simulink model "SystemLoopDiscrete2022"  (R2022b)
settings: Solver=FixedStepAuto  StartTime=0.0  StopTime=50  RelTol=1e-3  EnableMultiTasking=on
values from neighbouring files (symbols this model uses):
  L = 8.2*10^(-3)    (= 0.0082)    [phaseplane.m]
undefined symbols (not defined in the file or in its folder): Ad, Bd, Cd, Dd, ki, Kp, Ts
libraries: mbedblockslib x3, stm_qeplib x1
settings Model: ExtModeTrigDuration=10  Creator=Marco  LastModifiedBy=Marco
settings OptimizationCC: ReuseModelBlockBuffer=on  EnhancedBackFolding=on  PassReuseOutputArgsAs=Individual arguments  ZeroExternalMemoryAtStartup=off  ZeroInternalMemoryAtStartup=off  MaxStackSize=64  OptimizeBlockOrder=speed  DifferentSizesBufferReuse=on  OptimizationCustomize=off  EfficientTunableParamExpr=on
settings DebuggingCC: ParameterTunabilityLossMsg=error
settings HardwareCC: ProdBitPerPointer=32  ProdBitPerSizeT=32  ProdBitPerPtrDiffT=32  ProdLargestAtomicInteger=Long  ProdLargestAtomicFloat=Double  ProdWordSize=32  ProdLongLongMode=on  ProdHWDeviceType=ARM Compatible->ARM Cortex
settings SFSimCC: MATLABDynamicMemAlloc=off
settings RTWCC: Description=Embedded Coder  SystemTargetFile=ert.tlc  HardwareBoard=STM32 Nucleo F401RE  TemplateMakefile=ert_default_tmf  Toolchain=GNU Tools for ARM Embedded Processors
settings CodeAppCC: ForceParamTrailComments=on  IgnoreCustomStorageClasses=off  OperatorAnnotations=on  SimulinkDataObjDesc=on  SFDataObjDesc=on  InsertBlockDesc=on
settings ERTTargetCC: ExtMode=on  ExtModeTransport=3  ExtModeStaticAlloc=on  ExtModeStaticAllocSize=2000  ExtModeMexFile=ext_xcp  ExtModeMexArgs=1 3 115200  ExtModeIntrfLevel=Level2 - Open

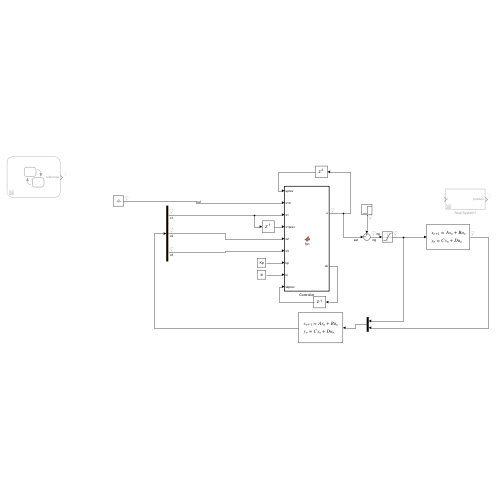
[thumbnail: Simulink's stored preview of the top-level diagram]
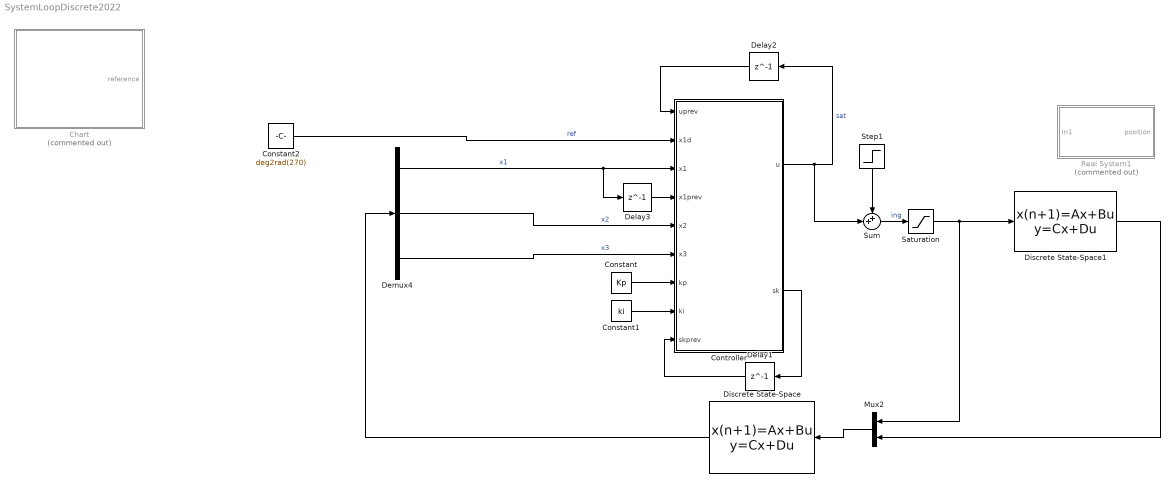
== system SystemLoopDiscrete2022 ==
  Chart : Stateflow chart  Commented=on  TreatAsAtomicUnit=on
  Constant : Constant  Value=Kp  SampleTime=Ts
  Constant1 : Constant  Value=ki  SampleTime=Ts
  Constant2 : Constant  Value=deg2rad(270)
  Controller : MATLAB Function  TreatAsAtomicUnit=on
  Delay1 : Delay  DelayLength=1  InitialCondition=0
  Delay2 : Delay  DelayLength=1  InitialCondition=0
  Delay3 : Delay  DelayLength=1  InitialCondition=0
  Demux4 : Demux  Outputs=3
  Discrete State-Space : DiscreteStateSpace  A=Ad-L*Cd  B=[Bd L]  C=eye(3)  D=[ 0 0; 0 0; 0 0]  SampleTime=Ts
  Discrete State-Space1 : DiscreteStateSpace  A=Ad  B=Bd  C=Cd  D=Dd  SampleTime=Ts
  Mux2 : Mux  Inputs=2
  Real System1 : Subsystem  Commented=on
  Saturation : Saturate  UpperLimit=12  LowerLimit=-12
  Step1 : Step  Time=3  After=1.2  SampleTime=Ts
  Sum : Sum  Inputs=++|
  wires:
  Discrete State-Space/1 -> Demux4/1
  Mux2/1 -> Discrete State-Space/1
  Demux4/2 -> Controller/5(x2)  "x2"
  Step1/1 -> Sum/1
  Sum/1 -> Saturation/1  "ing"
  Discrete State-Space1/1 -> Mux2/2
  Constant/1 -> Controller/7(kp)
  Constant2/1 -> Controller/2(x1d)  "ref"
  Demux4/1 -> Controller/3(x1), Delay3/1  "x1"
  Constant1/1 -> Controller/8(ki)
  Controller/1(u) -> Delay2/1, Sum/2  "sat"
  Demux4/3 -> Controller/6(x3)  "x3"
  Controller/2(sk) -> Delay1/1
  Delay1/1 -> Controller/9(skprev)
  Delay2/1 -> Controller/1(uprev)
  Delay3/1 -> Controller/4(x1prev)
  Saturation/1 -> Discrete State-Space1/1, Mux2/1

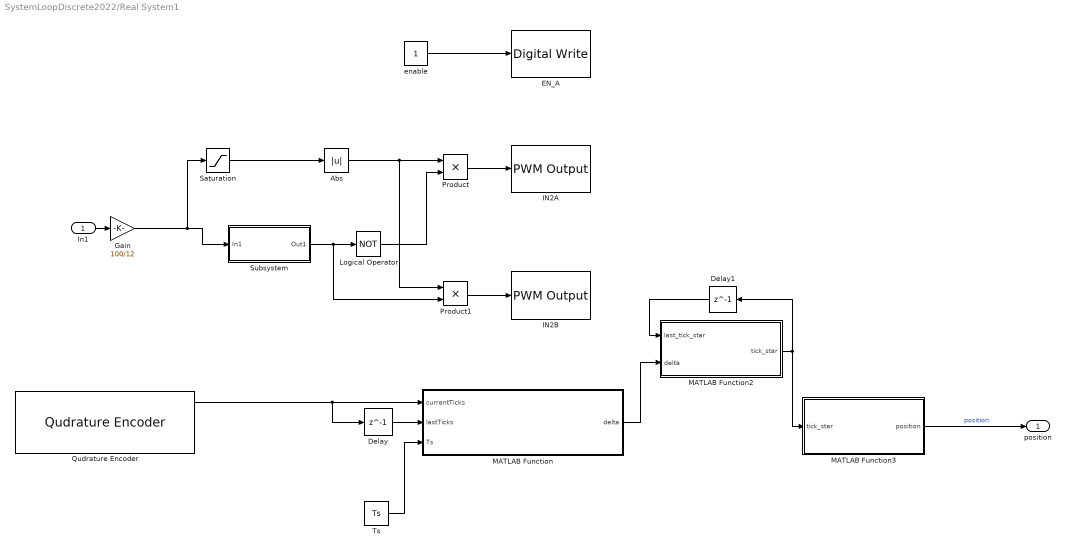
== system SystemLoopDiscrete2022/Real System1 ==
  In1 : Inport
  Abs : Abs  SaturateOnIntegerOverflow=off
  Delay : Delay  DelayLength=1  InitialCondition=0
  Delay1 : Delay  DelayLength=1  InitialCondition=0
  EN_A : mbedblockslib/Digital Write  Pin=2  Direction=output
      settings: LibrarySourceBlock=stmnucleorootlib/Common/Digital Write
  Gain : Gain  Gain=100/12
  IN2A : mbedblockslib/PWM Output  Pin=4  EnableInputFrequency=off  InitialFrequency=PWMFreq  InitialDutyCycle=50  NotificationType=None
      settings: LibrarySourceBlock=stmnucleorootlib/Common/PWM Output
  IN2B : mbedblockslib/PWM Output  Pin=5  EnableInputFrequency=off  InitialFrequency=PWMFreq  InitialDutyCycle=50  NotificationType=None
      settings: LibrarySourceBlock=stmnucleorootlib/Common/PWM Output
  Logical Operator : Logic  Operator=NOT  AllPortsSameDT=off  OutDataTypeStr=boolean
  MATLAB Function : MATLAB Function  TreatAsAtomicUnit=on
  MATLAB Function2 : MATLAB Function  TreatAsAtomicUnit=on
  MATLAB Function3 : MATLAB Function  TreatAsAtomicUnit=on
  Product : Product
  Product1 : Product
  Qudrature Encoder : stm_qeplib/Qudrature Encoder  SampleTime=Ts
  Saturation : Saturate  UpperLimit=100  LowerLimit=-100
  Subsystem : Subsystem
  Ts : Constant  Value=Ts
  enable : Constant
  position : Outport
  wires:
  enable/1 -> EN_A/1
  Subsystem/1(Out1) -> Product1/2, Logical Operator/1
  Saturation/1 -> Abs/1
  Product1/1 -> IN2B/1
  Product/1 -> IN2A/1
  Logical Operator/1 -> Product/2
  Abs/1 -> Product1/1, Product/1
  Gain/1 -> Saturation/1, Subsystem/1(In1)
  MATLAB Function2/1(tick_star) -> MATLAB Function3/1(tick_star), Delay1/1
  Qudrature Encoder/1 -> Delay/1, MATLAB Function/1(currentTicks)
  MATLAB Function/1(delta) -> MATLAB Function2/2(delta)
  Delay1/1 -> MATLAB Function2/1(last_tick_star)
  Ts/1 -> MATLAB Function/3(Ts)
  Delay/1 -> MATLAB Function/2(lastTicks)
  In1/1 -> Gain/1
  MATLAB Function3/1(position) -> position/1  "position"

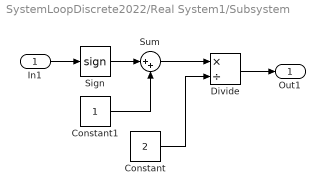
== system SystemLoopDiscrete2022/Real System1/Subsystem ==
  In1 : Inport
  Constant : Constant  Value=2
  Constant1 : Constant
  Divide : Product  Inputs=*/
  Sign : Signum
  Sum : Sum  Inputs=|++
  Out1 : Outport
  wires:
  In1/1 -> Sign/1
  Sign/1 -> Sum/1
  Constant1/1 -> Sum/2
  Sum/1 -> Divide/1
  Constant/1 -> Divide/2
  Divide/1 -> Out1/1

== stateflow chart SystemLoopDiscrete2022/Chart ==
  state Start
    reference = 0;
  state State1
    reference = deg2rad(180)
  state State4
    reference = -180
  state State2
    reference = deg2rad(360)
  state State3
    reference = deg2rad(270)
  state State5
    reference = 0
  (default) -> Start
  Start -> State1 : [after(4,sec)]
  State1 -> State4 : [after(4,sec)]
  State4 -> State2 : [after(4,sec)]
  State3 -> Start : [after(4,sec)]
  State2 -> State5 : [after(4,sec)]
  State5 -> State3 : [after(4,sec)]
  data: reference output

== matlab function SystemLoopDiscrete2022/Controller ==
  data: uprev input; x1d input; x1 input; x1prev input; u output; x2 input; x3 input; kp input; ki input; skprev input; sk output
function [u,sk] = fcn(uprev, x1d, x1, x1prev, x2, x3, kp, ki, skprev)

eprev = x1d-x1prev

stopsumm = ((uprev > 12 & eprev > 0) | (uprev < -12 & eprev < 0));

if ~(stopsumm)
   sk = skprev + eprev
   u = -kp(1)*(x1) - kp(2)*x2 - kp(3)*x3 + ki*sk;
else
   u = -kp(1)*(x1) - kp(2)*x2 - kp(3)*x3 + ki*skprev;
   sk = skprev
end

== matlab function SystemLoopDiscrete2022/Real System1/MATLAB Function ==
  data: currentTicks input; delta output; lastTicks input; Ts input
function delta = getTicksDelta(currentTicks, lastTicks, Ts)

currentTicks = double(currentTicks);
lastTicks = double(lastTicks);

if abs(currentTicks - lastTicks) <= ceil(8400*Ts)
    delta = currentTicks-lastTicks;
else
    if lastTicks > currentTicks
        delta = currentTicks + 2^16-1-lastTicks;
    else
        delta = currentTicks - 2^16+1-lastTicks;

end

end

== matlab function SystemLoopDiscrete2022/Real System1/MATLAB Function2 ==
  data: last_tick_star input; delta input; tick_star output
function tick_star = modCounter(last_tick_star, delta)

    % 89796 numero di tick per effettuare 25 giri completo
    tick_star = mod(last_tick_star + delta, 89796)

end

== matlab function SystemLoopDiscrete2022/Real System1/MATLAB Function3 ==
  data: tick_star input; position output
function position = getPosition(tick_star)

    tick_star = double(tick_star);

    completeTheta = 2*pi*tick_star/(3591.84);

    position = sign(completeTheta) * abs(completeTheta);

end
